simulink model "SSItest"  (R2020a)
settings: Solver=VariableStepAuto  StartTime=0.0  StopTime=1  RelTol=1e-3
undefined symbols (not defined in the file): D, E, Kgov, M, Pm, R, Tgov, Vr, wr, X
settings Model: Creator=EPESL  LastModifiedBy=EPESL
settings DataIOCC: ReturnWorkspaceOutputs=off
settings DebuggingCC: ArithmeticOperatorsInVariantConditions=warning
settings SFSimCC: CustomCodeUndefinedFunction=UseInterfaceOnly

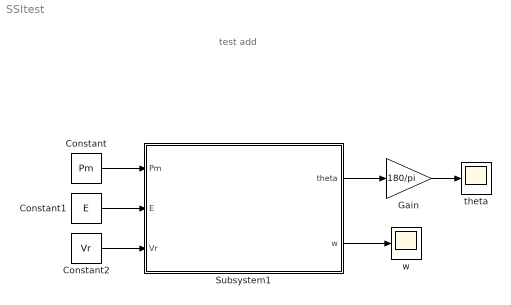
== system SSItest ==
  note: test add
  Constant : Constant  Value=Pm
  Constant1 : Constant  Value=E
  Constant2 : Constant  Value=Vr
  Gain : Gain  Gain=180/pi
  Subsystem1 : Subsystem
  theta : Scope
  w : Scope
  wires:
  Subsystem1/1(theta) -> Gain/1
  Subsystem1/2(w) -> w/1
  Constant/1 -> Subsystem1/1(Pm)
  Constant1/1 -> Subsystem1/2(E)
  Constant2/1 -> Subsystem1/3(Vr)
  Gain/1 -> theta/1

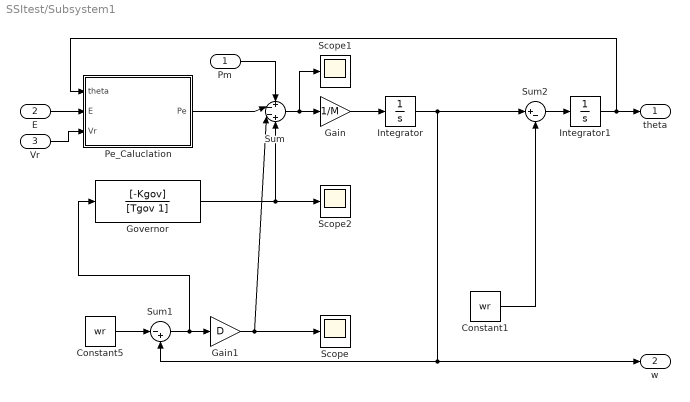
== system SSItest/Subsystem1 ==
  Pm : Inport
  E : Inport  Port=2
  Vr : Inport  Port=3
  Constant1 : Constant  Value=wr
  Constant5 : Constant  Value=wr
  Gain : Gain  Gain=1/M
  Gain1 : Gain  Gain=D
  Governor : TransferFcn  Numerator=[-Kgov]  Denominator=[Tgov 1]
  Integrator : Integrator  InitialCondition=2*pi*60
  Integrator1 : Integrator
  Pe_Caluclation : Subsystem
  Scope : Scope
  Scope1 : Scope
  Scope2 : Scope
  Sum : Sum  Inputs=+--+
  Sum1 : Sum  Inputs=|-+
  Sum2 : Sum  Inputs=|+-
  theta : Outport  VectorParamsAs1DForOutWhenUnconnected=off
  w : Outport  Port=2  VectorParamsAs1DForOutWhenUnconnected=off
  wires:
  Integrator/1 -> Sum2/1, Sum1/2, w/1
  Pe_Caluclation/1(Pe) -> Sum/2
  Sum1/1 -> Governor/1, Gain1/1
  Gain/1 -> Integrator/1
  Constant5/1 -> Sum1/1
  Sum/1 -> Scope1/1, Gain/1
  Gain1/1 -> Scope/1, Sum/3
  E/1 -> Pe_Caluclation/2(E)
  Integrator1/1 -> Pe_Caluclation/1(theta), theta/1
  Vr/1 -> Pe_Caluclation/3(Vr)
  Pm/1 -> Sum/1
  Sum2/1 -> Integrator1/1
  Constant1/1 -> Sum2/2
  Governor/1 -> Scope2/1, Sum/4

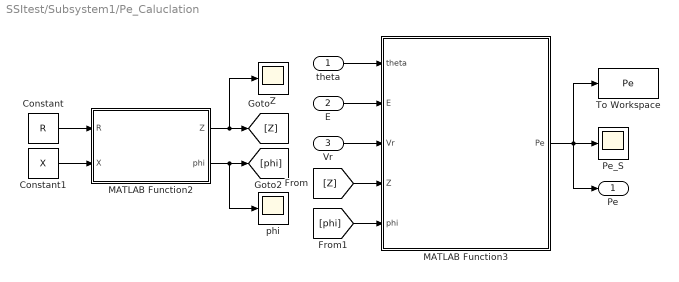
== system SSItest/Subsystem1/Pe_Caluclation ==
  theta : Inport
  E : Inport  Port=2
  Vr : Inport  Port=3
  Constant : Constant  Value=R
  Constant1 : Constant  Value=X
  MATLAB Function2 : MATLAB Function  TreatAsAtomicUnit=on
  MATLAB Function3 : MATLAB Function  TreatAsAtomicUnit=on
  Pe_S : Scope
  To Workspace : ToWorkspace  VariableName=Pe  SaveFormat=Timeseries  SampleTime=-1
  Z : Scope
  phi : Scope
  Pe : Outport  VectorParamsAs1DForOutWhenUnconnected=off
  wires:
  MATLAB Function3/1(Pe) -> To Workspace/1, Pe/1, Pe_S/1
  Constant/1 -> MATLAB Function2/1(R)
  Constant1/1 -> MATLAB Function2/2(X)
  [phi] -> MATLAB Function3/5(phi)
  [Z] -> MATLAB Function3/4(Z)
  Vr/1 -> MATLAB Function3/3(Vr)
  E/1 -> MATLAB Function3/2(E)
  theta/1 -> MATLAB Function3/1(theta)
  MATLAB Function2/2(phi) -> phi/1, [phi]
  MATLAB Function2/1(Z) -> Z/1, [Z]

== matlab function SSItest/Subsystem1/Pe_Caluclation/MATLAB Function3 ==
  data: theta input; E input; Vr input; Z input; phi input; Pe output
function Pe   = Func(theta, E, Vr, Z, phi)

Pe = ((E * Vr) / Z) * cos(phi - theta) - ((Vr^2) / Z) * cos(phi);
% Pe = ((E * Vr) / Z) * sin(theta);

== matlab function SSItest/Subsystem1/Pe_Caluclation/MATLAB Function2 ==
  data: R input; Z output; X input; phi output
function [Z, phi]  = Func(R, X)
Z = sqrt(R^2 + X^2);
phi = atan(X / R);
